simulink model "Solar_Panel_control_system"  (R2024a)
settings: Solver=VariableStepAuto  StartTime=0.0  StopTime=15*3600  RelTol=1e-3
undefined symbols (not defined in the file): J, kd, Kf, Kg, Kt, L, R
libraries: slpidlib x1
settings Model: Creator=prat  LastModifiedBy=prat
settings DataIOCC: ExternalInput=[sunTime, sunPosition]  LoadExternalInput=on

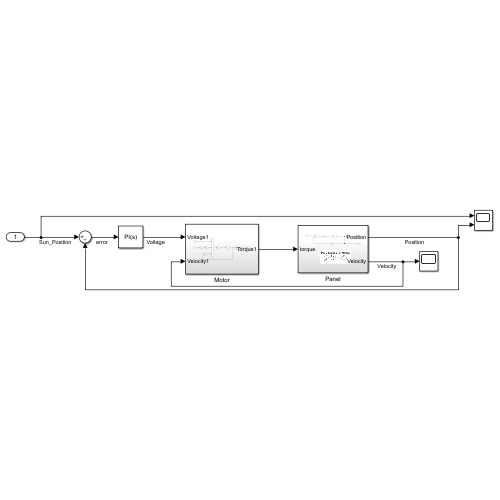
[thumbnail: Simulink's stored preview of the top-level diagram]
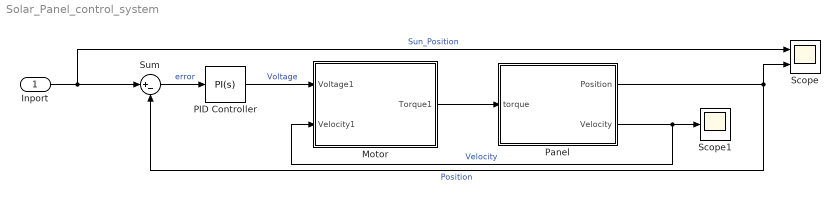
== system Solar_Panel_control_system ==
  Inport : Inport
  Motor : Subsystem
  PID Controller : slpidlib/PID Controller  Controller=PI  Form=Parallel  TimeDomain=Continuous-time  UseExternalTs=off  SampleTime=-1  IntegratorMethod=Forward Euler  FilterMethod=Forward Euler  ControllerParametersSource=internal  P=240  I=180  UseKiTs=off  D=0  UseExternalDerivativeSource=off  N=100  UseFilter=on  TunerSelectOption=Transfer Function Based (PID Tuner App)  InitialConditionSource=internal  InitialConditionForIntegrator=0  InitialConditionForFilter=0  DifferentiatorICPrevScaledInput=0  ExternalReset=none  TrackingMode=off  Kt=1  LimitOutput=off  SatLimitsSource=internal  UpperSaturationLimit=inf  LowerSaturationLimit=-inf  LinearizeAsGain=on  AntiWindupMode=none  Kb=1  LimitIntegrator=off  UpperIntegratorSaturationLimit=inf  LowerIntegratorSaturationLimit=-inf  POutMin=[]  POutMax=[]  IOutMin=[]  IOutMax=[]  DOutMin=[]  DOutMax=[]  NOutMin=[]  NOutMax=[]  SumOutMin=[]  SumOutMax=[]  SaturationOutMin=[]  SaturationOutMax=[]  PParamMin=[]  PParamMax=[]  IParamMin=[]  IParamMax=[]  DParamMin=[]  DParamMax=[]  NParamMin=[]  NParamMax=[]  KbParamMin=[]  KbParamMax=[]  KtParamMin=[]  KtParamMax=[]  KbOutMin=[]  KbOutMax=[]  KtOutMin=[]  KtOutMax=[]  IntegratorOutMin=[]  IntegratorOutMax=[]  FilterOutMin=[]  FilterOutMax=[]  SumI1OutMin=[]  SumI1OutMax=[]  SumI2OutMin=[]  SumI2OutMax=[]  SumI3OutMin=[]  SumI3OutMax=[]  SumI4OutMin=[]  SumI4OutMax=[]  SumDOutMin=[]  SumDOutMax=[]  DifferentiatorOutMin=[]  DifferentiatorOutMax=[]  FilterDiffOutCoefMin=[]  FilterDiffOutCoefMax=[]  ReciprocalOutMin=[]  ReciprocalOutMax=[]  SumDenOutMin=[]  SumDenOutMax=[]  SumNumOutMin=[]  SumNumOutMax=[]  DivideOutMin=[]  DivideOutMax=[]  UdiffTsProdOutMin=[]  UdiffTsProdOutMax=[]  NTsProdOutMin=[]  NTsProdOutMax=[]  UintegralTsProdOutMin=[]  UintegralTsProdOutMax=[]  UngainTsProdOutMin=[]  UngainTsProdOutMax=[]  ClampingZeroOutDataTypeStr=Inherit: Inherit via back propagation  ClampingZeroOutMin=[]  ClampingZeroOutMax=[]  FilterDenConstantOutDataTypeStr=Inherit: Inherit via back propagation  FilterDenConstantOutMin=[]  FilterDenConstantOutMax=[]  PCopyOutDataTypeStr=Inherit: Inherit via back propagation  PCopyOutMin=[]  PCopyOutMax=[]  NCopyOutDataTypeStr=Inherit: Inherit via back propagation  NCopyOutMin=[]  NCopyOutMax=[]  IntegratorContinuousStateAttributes=''  IntegratorStateMustResolveToSignalObject=off  IntegratorRTWStateStorageClass=Auto  FilterContinuousStateAttributes=''  FilterStateMustResolveToSignalObject=off  FilterRTWStateStorageClass=Auto  ParallelPVariant=InternalParameters  IdealPVariant=Disabled  IVariant=InternalParameters  DVariant=Disabled  IntegratorVariant=Continuous  SatVariant=Disabled  AWVariant=Passthrough  PCopyVariant=Disabled  TRVariant=Disabled  FdbkBlocksVariant=Forward  IdealPFdbkVariant=Disabled  SatFdbkVariant=Disabled  DerivativeFilterVariant=Disabled  NVariant=Disabled  NCopyVariant=Disabled_SignalSpec  FilterICVariant=Disabled  IntegratorICVariant=InternalICs  ExternalResetVariant=Disabled  TRSumVariant=Passthrough  SumFdbkVariant=Disabled  SumVariant=Sum_PI  TsampFilterVariant=InternalTs  TsampNgainVariant=Passthrough  TsampIntegralVariant=Disabled_SignalSpec  ExternalSaturationOutDataTypeStr=Inherit: Same as second input  DerivativeSourceVariant=Disabled
  Panel : Subsystem
  Scope : Scope  NumInputPorts=2
  Scope1 : Scope
  Sum : Sum  Inputs=|+-
  wires:
  Panel/1(Position) -> Sum/2, Scope/2  "Position"
  Panel/2(Velocity) -> Motor/2(Velocity1), Scope1/1  "Velocity"
  Sum/1 -> PID Controller/1  "error"
  Inport/1 -> Scope/1, Sum/1  "Sun_Position"
  PID Controller/1 -> Motor/1(Voltage1)  "Voltage"
  Motor/1(Torque1) -> Panel/1(torque)

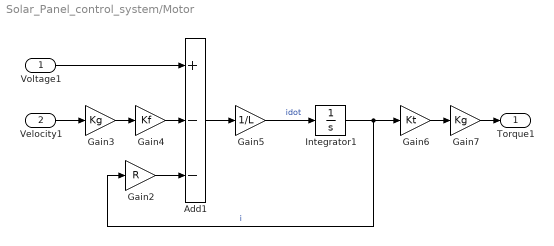
== system Solar_Panel_control_system/Motor ==
  Voltage1 : Inport
  Velocity1 : Inport  Port=2
  Add1 : Sum  Inputs=+--
  Gain2 : Gain  Gain=R
  Gain3 : Gain  Gain=Kg
  Gain4 : Gain  Gain=Kf
  Gain5 : Gain  Gain=1/L
  Gain6 : Gain  Gain=Kt
  Gain7 : Gain  Gain=Kg
  Integrator1 : Integrator
  Torque1 : Outport
  wires:
  Add1/1 -> Gain5/1
  Gain6/1 -> Gain7/1
  Gain3/1 -> Gain4/1
  Integrator1/1 -> Gain6/1, Gain2/1  "i"
  Velocity1/1 -> Gain3/1
  Gain7/1 -> Torque1/1
  Gain5/1 -> Integrator1/1  "idot"
  Voltage1/1 -> Add1/1
  Gain2/1 -> Add1/3
  Gain4/1 -> Add1/2

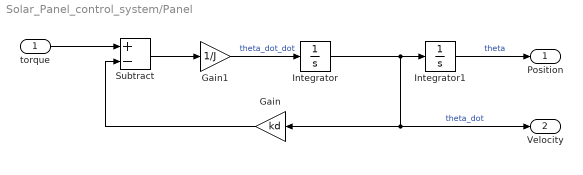
== system Solar_Panel_control_system/Panel ==
  torque : Inport
  Gain : Gain  Gain=kd
  Gain1 : Gain  Gain=1/J
  Integrator : Integrator
  Integrator1 : Integrator
  Subtract : Sum  Inputs=+-
  Position : Outport
  Velocity : Outport  Port=2
  wires:
  Subtract/1 -> Gain1/1
  Integrator/1 -> Velocity/1, Gain/1, Integrator1/1  "theta_dot"
  Gain/1 -> Subtract/2
  Gain1/1 -> Integrator/1  "theta_dot_dot"
  Integrator1/1 -> Position/1  "theta"
  torque/1 -> Subtract/1
